simulink model "gm_uz_mlp_three_layer"  (R2021a)
settings: Solver=FixedStepDiscrete  StartTime=0.0  StopTime=5000  RelTol=1e-3
undefined symbols (not defined in the file or in its folder): nn, nn_data_type_max, numInput, numOut
libraries: hdlsllib x94, simulink x85
(part 3 of 4)

== system gm_uz_mlp_three_layer/uz_mlp_three_layer/reluLayer_8Parallel/MAC7 ==
  rd_addr : Inport  OutDataTypeStr=fixdt(0, 10, 0)  PortDimensions=1  SampleTime=1
  b : Inport  Port=2  OutDataTypeStr=fixdt(1, 32, 14)  PortDimensions=1  SampleTime=1
  axi_signals : Inport  Port=3  SampleTime=1
  fromStateMachine : Inport  Port=4  SampleTime=1
  AND : Logic  IconShape=distinctive  AllPortsSameDT=off  OutDataTypeStr=boolean
  AND1 : Logic  IconShape=distinctive  AllPortsSameDT=off  OutDataTypeStr=boolean
  Bus Selector : BusSelector  OutputSignals=axi_weightData,axi_weightAddr,axi_weightsWriteEnable,axi_biasData,axi_biasAddr,axi_biasWriteEnable,axi_layerNr
  Bus Selector1 : BusSelector  OutputSignals=endin,validIn,startin,mac_counter,write_enable,n_perceptron
  Compare To Constant : simulink/Logic and Bit Operations/Compare To Constant  relop===  const=ParallelNr  OutDataTypeStr=boolean
  Compare To Constant1 : simulink/Logic and Bit Operations/Compare To Constant  relop===  const=ParallelNr  OutDataTypeStr=boolean
  Compare To Constant2 : simulink/Logic and Bit Operations/Compare To Constant  relop===  const=LayerNr  OutDataTypeStr=boolean
  Constant : Constant  Value=nStart  OutDataTypeStr=Inherit: Inherit via back propagation  SampleTime=-1
  Dual Port RAM System1 : hdlsllib/HDL RAMs/Dual Port RAM System  RAMType=Simple dual port  WriteOutputValue=New data  RAMInitialValue=[layer.bias(nStart:nEnd);zeros(1024-length(layer.bias(nStart:nEnd)),1)]  SimulateUsing=Code generation
      settings: SourceProductBaseCode=SL
  Dual Port RAM System2 : hdlsllib/HDL RAMs/Dual Port RAM System  RAMType=Simple dual port  WriteOutputValue=New data  RAMInitialValue=[0]  SimulateUsing=Code generation
      settings: SourceProductBaseCode=SL
  Dual Port RAM System3 : hdlsllib/HDL RAMs/Dual Port RAM System  RAMType=Simple dual port  WriteOutputValue=New data  RAMInitialValue=[0;reshape(layer.weights(:,nStart:nEnd),[],1);zeros(1023-length(reshape(layer.weights(:,nStart:nEnd),[],1)),1)]  SimulateUsing=Code generation
      settings: SourceProductBaseCode=SL
  Gain : Gain  Gain=size(layer.weights(:,nStart:nEnd),1)  OutDataTypeStr=Inherit: Same as input
  Multiply-Accumulate1 : hdlsllib/HDL Operations/Multiply-Accumulate  opMode=Streaming - using Start and End ports  initValueSetting=Dialog  initValue=0  initValueSetting2=Input port  initValue2=0  initValueSetting3=Dialog  initValue3=0  num_samples=2  RndMeth2=Floor  RndMeth3=Floor  datatype2=fixdt(1,32,14)  datatype3=Inherit: Inherit via back propagation  validOut=on  endInandOut=on  startOut=on  countOut=on  dim=-1  DoSatur=off  parallel=off
      settings: SourceProductBaseCode=SL
  Saturation1 : Saturate  UpperLimit=nn_data_type_max  LowerLimit=0
  Sum : Sum  Inputs=|++  OutDataTypeStr=Inherit: Same as first input
  Sum1 : Sum  Inputs=|++  OutDataTypeStr=Inherit: Same as first input
  Terminator : Terminator
  rd_dout : Outport  SampleTime=1
  startOut : Outport  Port=2  SampleTime=1
  endOut : Outport  Port=3  SampleTime=1
  wires:
  rd_addr/1 -> Dual Port RAM System2/4
  b/1 -> Multiply-Accumulate1/2
  axi_signals/1 -> Bus Selector/1
  fromStateMachine/1 -> Bus Selector1/1
  AND/1 -> Dual Port RAM System3/3
  AND1/1 -> Dual Port RAM System1/3
  Bus Selector/1 -> Dual Port RAM System3/1
  Bus Selector/2 -> Dual Port RAM System3/2
  Bus Selector/3 -> Compare To Constant/1
  Bus Selector/4 -> Dual Port RAM System1/1
  Bus Selector/5 -> Dual Port RAM System1/2
  Bus Selector/6 -> Compare To Constant1/1
  Bus Selector/7 -> Compare To Constant2/1
  Bus Selector1/1 -> Multiply-Accumulate1/4
  Bus Selector1/2 -> Multiply-Accumulate1/5
  Bus Selector1/3 -> Multiply-Accumulate1/3
  Bus Selector1/4 -> Sum1/2
  Bus Selector1/5 -> Dual Port RAM System2/3
  Bus Selector1/6 -> Sum/1, Gain/1, Dual Port RAM System1/4
  Compare To Constant/1 -> AND/1
  Compare To Constant1/1 -> AND1/1
  Compare To Constant2/1 -> AND1/2, AND/2
  Constant/1 -> Sum/2
  Dual Port RAM System1/1 -> Multiply-Accumulate1/6
  Dual Port RAM System2/1 -> rd_dout/1
  Dual Port RAM System3/1 -> Multiply-Accumulate1/1
  Gain/1 -> Sum1/1
  Multiply-Accumulate1/1 -> Saturation1/1
  Multiply-Accumulate1/2 -> startOut/1
  Multiply-Accumulate1/3 -> endOut/1
  Multiply-Accumulate1/4 -> Terminator/1
  Saturation1/1 -> Dual Port RAM System2/1
  Sum/1 -> Dual Port RAM System2/2
  Sum1/1 -> Dual Port RAM System3/4

== system gm_uz_mlp_three_layer/uz_mlp_three_layer/reluLayer_8Parallel/MATLAB Function1 ==
  readAddr : Inport  OutDataTypeStr=fixdt(0, 10, 0)  PortDimensions=1  SampleTime=1
  MATLAB Function1 : MATLAB Function  TreatAsAtomicUnit=on
  y : Outport  SampleTime=1
  wires:
  readAddr/1 -> MATLAB Function1/1(readAddr)
  MATLAB Function1/1(y) -> y/1

== system gm_uz_mlp_three_layer/uz_mlp_three_layer/reluLayer_8Parallel/StateMachines1 ==
  triggerCalc : Inport  OutDataTypeStr=boolean  SampleTime=1
  mac_startOut : Inport  Port=2  OutDataTypeStr=boolean  SampleTime=1
  end_out : Inport  Port=3  OutDataTypeStr=boolean  SampleTime=1
  Bus Creator : BusCreator  Inputs=6
  Compare To Constant : simulink/Logic and Bit Operations/Compare To Constant  relop===  const=layer.weight_dimension(1)  OutDataTypeStr=boolean
  Compare To Constant1 : simulink/Logic and Bit Operations/Compare To Constant  relop===  const=layer.weight_dimension(2)/ParallelDSP-1  OutDataTypeStr=boolean
  Delay2 : Delay  DelayLength=1
  Delay3 : Delay  DelayLength=1
  Delay4 : Delay  DelayLength=1
  Detect Rise Positive : simulink/Logic and Bit Operations/Detect Rise Positive  vinit=0  OutDataTypeStr=boolean
  index_counter : hdlsllib/Sources/HDL Counter  CountType=Count limited  CountInit=1  CountStep=1  CountMax=layer.weight_dimension(1)  CountFromType=Initial value  CountFrom=1  CountResetPort=on  CountLoadPort=off  CountEnbPort=on  CountDirPort=off  CountHitOutputPort=off  CountDataType=Unsigned  CountWordLen=10  CountFracLen=0  CountSampTime=1
  layer_control : Subsystem
  mac_control : Subsystem
  perceptron_counter1 : hdlsllib/Sources/HDL Counter  CountType=Count limited  CountInit=0  CountStep=1  CountMax=layer.weight_dimension(2)/ParallelDSP-1  CountFromType=Initial value  CountFrom=0  CountResetPort=on  CountLoadPort=off  CountEnbPort=on  CountDirPort=off  CountHitOutputPort=off  CountDataType=Unsigned  CountWordLen=10  CountFracLen=0  CountSampTime=1
  mac_counter : Outport  SampleTime=1
  layer_rdy : Outport  Port=2  SampleTime=1
  layer_finished : Outport  Port=3  SampleTime=1
  toMac : Outport  Port=4  SampleTime=1
  wires:
  triggerCalc/1 -> Detect Rise Positive/1
  mac_startOut/1 -> mac_control/5(mac_startOut)
  end_out/1 -> Delay3/1, mac_control/3(end_out)
  Bus Creator/1 -> toMac/1
  Compare To Constant/1 -> mac_control/2(counter_finished)
  Compare To Constant1/1 -> layer_control/3(cnt_finished)
  Delay2/1 -> Compare To Constant/1
  Delay3/1 -> mac_control/4(end_out_delay)
  Delay4/1 -> layer_control/2(mac_ready)
  Detect Rise Positive/1 -> layer_control/1(ext_enable)
  index_counter/1 -> Bus Creator/4, Delay2/1, mac_counter/1  "mac_counter"
  layer_control/1(enable_mac) -> mac_control/1(external_enable)
  layer_control/2(layer_rdy) -> layer_rdy/1
  layer_control/3(cnt_enable) -> perceptron_counter1/2
  layer_control/4(counter_rest) -> perceptron_counter1/1
  layer_control/5(layer_finished) -> layer_finished/1
  mac_control/1(index_counter_enb) -> index_counter/2
  mac_control/2(mac_startIn) -> Bus Creator/3  "startin"
  mac_control/3(mac_endIn) -> Bus Creator/1  "endin"
  mac_control/4(mac_validIn) -> Bus Creator/2  "validIn"
  mac_control/5(index_counter_rst) -> index_counter/1
  mac_control/6(write_ram) -> Bus Creator/5  "write_enable"
  mac_control/7(mac_ready) -> Delay4/1
  perceptron_counter1/1 -> Compare To Constant1/1, Bus Creator/6  "n_perceptron"

== system gm_uz_mlp_three_layer/uz_mlp_three_layer/reluLayer_8Parallel1/MAC ==
  rd_addr : Inport  OutDataTypeStr=fixdt(0, 10, 0)  PortDimensions=1  SampleTime=1
  b : Inport  Port=2  OutDataTypeStr=fixdt(1, 32, 14)  PortDimensions=1  SampleTime=1
  axi_signals : Inport  Port=3  SampleTime=1
  fromStateMachine : Inport  Port=4  SampleTime=1
  AND : Logic  IconShape=distinctive  AllPortsSameDT=off  OutDataTypeStr=boolean
  AND1 : Logic  IconShape=distinctive  AllPortsSameDT=off  OutDataTypeStr=boolean
  Bus Selector : BusSelector  OutputSignals=axi_weightData,axi_weightAddr,axi_weightsWriteEnable,axi_biasData,axi_biasAddr,axi_biasWriteEnable,axi_layerNr
  Bus Selector1 : BusSelector  OutputSignals=endin,validIn,startin,mac_counter,write_enable,n_perceptron
  Compare To Constant : simulink/Logic and Bit Operations/Compare To Constant  relop===  const=ParallelNr  OutDataTypeStr=boolean
  Compare To Constant1 : simulink/Logic and Bit Operations/Compare To Constant  relop===  const=ParallelNr  OutDataTypeStr=boolean
  Compare To Constant2 : simulink/Logic and Bit Operations/Compare To Constant  relop===  const=LayerNr  OutDataTypeStr=boolean
  Constant : Constant  Value=nStart  OutDataTypeStr=Inherit: Inherit via back propagation  SampleTime=-1
  Dual Port RAM System1 : hdlsllib/HDL RAMs/Dual Port RAM System  RAMType=Simple dual port  WriteOutputValue=New data  RAMInitialValue=[layer.bias(nStart:nEnd);zeros(1024-length(layer.bias(nStart:nEnd)),1)]  SimulateUsing=Code generation
      settings: SourceProductBaseCode=SL
  Dual Port RAM System2 : hdlsllib/HDL RAMs/Dual Port RAM System  RAMType=Simple dual port  WriteOutputValue=New data  RAMInitialValue=[0]  SimulateUsing=Code generation
      settings: SourceProductBaseCode=SL
  Dual Port RAM System3 : hdlsllib/HDL RAMs/Dual Port RAM System  RAMType=Simple dual port  WriteOutputValue=New data  RAMInitialValue=[0;reshape(layer.weights(:,nStart:nEnd),[],1);zeros(1023-length(reshape(layer.weights(:,nStart:nEnd),[],1)),1)]  SimulateUsing=Code generation
      settings: SourceProductBaseCode=SL
  Gain : Gain  Gain=size(layer.weights(:,nStart:nEnd),1)  OutDataTypeStr=Inherit: Same as input
  Multiply-Accumulate1 : hdlsllib/HDL Operations/Multiply-Accumulate  opMode=Streaming - using Start and End ports  initValueSetting=Dialog  initValue=0  initValueSetting2=Input port  initValue2=0  initValueSetting3=Dialog  initValue3=0  num_samples=2  RndMeth2=Floor  RndMeth3=Floor  datatype2=fixdt(1,32,14)  datatype3=Inherit: Inherit via back propagation  validOut=on  endInandOut=on  startOut=on  countOut=on  dim=-1  DoSatur=off  parallel=off
      settings: SourceProductBaseCode=SL
  Saturation1 : Saturate  UpperLimit=nn_data_type_max  LowerLimit=0
  Sum : Sum  Inputs=|++  OutDataTypeStr=Inherit: Same as first input
  Sum1 : Sum  Inputs=|++  OutDataTypeStr=Inherit: Same as first input
  Terminator : Terminator
  rd_dout : Outport  SampleTime=1
  startOut : Outport  Port=2  SampleTime=1
  endOut : Outport  Port=3  SampleTime=1
  wires:
  rd_addr/1 -> Dual Port RAM System2/4
  b/1 -> Multiply-Accumulate1/2
  axi_signals/1 -> Bus Selector/1
  fromStateMachine/1 -> Bus Selector1/1
  AND/1 -> Dual Port RAM System3/3
  AND1/1 -> Dual Port RAM System1/3
  Bus Selector/1 -> Dual Port RAM System3/1
  Bus Selector/2 -> Dual Port RAM System3/2
  Bus Selector/3 -> Compare To Constant/1
  Bus Selector/4 -> Dual Port RAM System1/1
  Bus Selector/5 -> Dual Port RAM System1/2
  Bus Selector/6 -> Compare To Constant1/1
  Bus Selector/7 -> Compare To Constant2/1
  Bus Selector1/1 -> Multiply-Accumulate1/4
  Bus Selector1/2 -> Multiply-Accumulate1/5
  Bus Selector1/3 -> Multiply-Accumulate1/3
  Bus Selector1/4 -> Sum1/2
  Bus Selector1/5 -> Dual Port RAM System2/3
  Bus Selector1/6 -> Sum/1, Gain/1, Dual Port RAM System1/4
  Compare To Constant/1 -> AND/1
  Compare To Constant1/1 -> AND1/1
  Compare To Constant2/1 -> AND1/2, AND/2
  Constant/1 -> Sum/2
  Dual Port RAM System1/1 -> Multiply-Accumulate1/6
  Dual Port RAM System2/1 -> rd_dout/1
  Dual Port RAM System3/1 -> Multiply-Accumulate1/1
  Gain/1 -> Sum1/1
  Multiply-Accumulate1/1 -> Saturation1/1
  Multiply-Accumulate1/2 -> startOut/1
  Multiply-Accumulate1/3 -> endOut/1
  Multiply-Accumulate1/4 -> Terminator/1
  Saturation1/1 -> Dual Port RAM System2/1
  Sum/1 -> Dual Port RAM System2/2
  Sum1/1 -> Dual Port RAM System3/4

== system gm_uz_mlp_three_layer/uz_mlp_three_layer/reluLayer_8Parallel1/MAC1 ==
  rd_addr : Inport  OutDataTypeStr=fixdt(0, 10, 0)  PortDimensions=1  SampleTime=1
  b : Inport  Port=2  OutDataTypeStr=fixdt(1, 32, 14)  PortDimensions=1  SampleTime=1
  axi_signals : Inport  Port=3  SampleTime=1
  fromStateMachine : Inport  Port=4  SampleTime=1
  AND : Logic  IconShape=distinctive  AllPortsSameDT=off  OutDataTypeStr=boolean
  AND1 : Logic  IconShape=distinctive  AllPortsSameDT=off  OutDataTypeStr=boolean
  Bus Selector : BusSelector  OutputSignals=axi_weightData,axi_weightAddr,axi_weightsWriteEnable,axi_biasData,axi_biasAddr,axi_biasWriteEnable,axi_layerNr
  Bus Selector1 : BusSelector  OutputSignals=endin,validIn,startin,mac_counter,write_enable,n_perceptron
  Compare To Constant : simulink/Logic and Bit Operations/Compare To Constant  relop===  const=ParallelNr  OutDataTypeStr=boolean
  Compare To Constant1 : simulink/Logic and Bit Operations/Compare To Constant  relop===  const=ParallelNr  OutDataTypeStr=boolean
  Compare To Constant2 : simulink/Logic and Bit Operations/Compare To Constant  relop===  const=LayerNr  OutDataTypeStr=boolean
  Constant : Constant  Value=nStart  OutDataTypeStr=Inherit: Inherit via back propagation  SampleTime=-1
  Dual Port RAM System1 : hdlsllib/HDL RAMs/Dual Port RAM System  RAMType=Simple dual port  WriteOutputValue=New data  RAMInitialValue=[layer.bias(nStart:nEnd);zeros(1024-length(layer.bias(nStart:nEnd)),1)]  SimulateUsing=Code generation
      settings: SourceProductBaseCode=SL
  Dual Port RAM System2 : hdlsllib/HDL RAMs/Dual Port RAM System  RAMType=Simple dual port  WriteOutputValue=New data  RAMInitialValue=[0]  SimulateUsing=Code generation
      settings: SourceProductBaseCode=SL
  Dual Port RAM System3 : hdlsllib/HDL RAMs/Dual Port RAM System  RAMType=Simple dual port  WriteOutputValue=New data  RAMInitialValue=[0;reshape(layer.weights(:,nStart:nEnd),[],1);zeros(1023-length(reshape(layer.weights(:,nStart:nEnd),[],1)),1)]  SimulateUsing=Code generation
      settings: SourceProductBaseCode=SL
  Gain : Gain  Gain=size(layer.weights(:,nStart:nEnd),1)  OutDataTypeStr=Inherit: Same as input
  Multiply-Accumulate1 : hdlsllib/HDL Operations/Multiply-Accumulate  opMode=Streaming - using Start and End ports  initValueSetting=Dialog  initValue=0  initValueSetting2=Input port  initValue2=0  initValueSetting3=Dialog  initValue3=0  num_samples=2  RndMeth2=Floor  RndMeth3=Floor  datatype2=fixdt(1,32,14)  datatype3=Inherit: Inherit via back propagation  validOut=on  endInandOut=on  startOut=on  countOut=on  dim=-1  DoSatur=off  parallel=off
      settings: SourceProductBaseCode=SL
  Saturation1 : Saturate  UpperLimit=nn_data_type_max  LowerLimit=0
  Sum : Sum  Inputs=|++  OutDataTypeStr=Inherit: Same as first input
  Sum1 : Sum  Inputs=|++  OutDataTypeStr=Inherit: Same as first input
  Terminator : Terminator
  rd_dout : Outport  SampleTime=1
  startOut : Outport  Port=2  SampleTime=1
  endOut : Outport  Port=3  SampleTime=1
  wires:
  rd_addr/1 -> Dual Port RAM System2/4
  b/1 -> Multiply-Accumulate1/2
  axi_signals/1 -> Bus Selector/1
  fromStateMachine/1 -> Bus Selector1/1
  AND/1 -> Dual Port RAM System3/3
  AND1/1 -> Dual Port RAM System1/3
  Bus Selector/1 -> Dual Port RAM System3/1
  Bus Selector/2 -> Dual Port RAM System3/2
  Bus Selector/3 -> Compare To Constant/1
  Bus Selector/4 -> Dual Port RAM System1/1
  Bus Selector/5 -> Dual Port RAM System1/2
  Bus Selector/6 -> Compare To Constant1/1
  Bus Selector/7 -> Compare To Constant2/1
  Bus Selector1/1 -> Multiply-Accumulate1/4
  Bus Selector1/2 -> Multiply-Accumulate1/5
  Bus Selector1/3 -> Multiply-Accumulate1/3
  Bus Selector1/4 -> Sum1/2
  Bus Selector1/5 -> Dual Port RAM System2/3
  Bus Selector1/6 -> Sum/1, Gain/1, Dual Port RAM System1/4
  Compare To Constant/1 -> AND/1
  Compare To Constant1/1 -> AND1/1
  Compare To Constant2/1 -> AND1/2, AND/2
  Constant/1 -> Sum/2
  Dual Port RAM System1/1 -> Multiply-Accumulate1/6
  Dual Port RAM System2/1 -> rd_dout/1
  Dual Port RAM System3/1 -> Multiply-Accumulate1/1
  Gain/1 -> Sum1/1
  Multiply-Accumulate1/1 -> Saturation1/1
  Multiply-Accumulate1/2 -> startOut/1
  Multiply-Accumulate1/3 -> endOut/1
  Multiply-Accumulate1/4 -> Terminator/1
  Saturation1/1 -> Dual Port RAM System2/1
  Sum/1 -> Dual Port RAM System2/2
  Sum1/1 -> Dual Port RAM System3/4

== system gm_uz_mlp_three_layer/uz_mlp_three_layer/reluLayer_8Parallel1/MAC2 ==
  rd_addr : Inport  OutDataTypeStr=fixdt(0, 10, 0)  PortDimensions=1  SampleTime=1
  b : Inport  Port=2  OutDataTypeStr=fixdt(1, 32, 14)  PortDimensions=1  SampleTime=1
  axi_signals : Inport  Port=3  SampleTime=1
  fromStateMachine : Inport  Port=4  SampleTime=1
  AND : Logic  IconShape=distinctive  AllPortsSameDT=off  OutDataTypeStr=boolean
  AND1 : Logic  IconShape=distinctive  AllPortsSameDT=off  OutDataTypeStr=boolean
  Bus Selector : BusSelector  OutputSignals=axi_weightData,axi_weightAddr,axi_weightsWriteEnable,axi_biasData,axi_biasAddr,axi_biasWriteEnable,axi_layerNr
  Bus Selector1 : BusSelector  OutputSignals=endin,validIn,startin,mac_counter,write_enable,n_perceptron
  Compare To Constant : simulink/Logic and Bit Operations/Compare To Constant  relop===  const=ParallelNr  OutDataTypeStr=boolean
  Compare To Constant1 : simulink/Logic and Bit Operations/Compare To Constant  relop===  const=ParallelNr  OutDataTypeStr=boolean
  Compare To Constant2 : simulink/Logic and Bit Operations/Compare To Constant  relop===  const=LayerNr  OutDataTypeStr=boolean
  Constant : Constant  Value=nStart  OutDataTypeStr=Inherit: Inherit via back propagation  SampleTime=-1
  Dual Port RAM System1 : hdlsllib/HDL RAMs/Dual Port RAM System  RAMType=Simple dual port  WriteOutputValue=New data  RAMInitialValue=[layer.bias(nStart:nEnd);zeros(1024-length(layer.bias(nStart:nEnd)),1)]  SimulateUsing=Code generation
      settings: SourceProductBaseCode=SL
  Dual Port RAM System2 : hdlsllib/HDL RAMs/Dual Port RAM System  RAMType=Simple dual port  WriteOutputValue=New data  RAMInitialValue=[0]  SimulateUsing=Code generation
      settings: SourceProductBaseCode=SL
  Dual Port RAM System3 : hdlsllib/HDL RAMs/Dual Port RAM System  RAMType=Simple dual port  WriteOutputValue=New data  RAMInitialValue=[0;reshape(layer.weights(:,nStart:nEnd),[],1);zeros(1023-length(reshape(layer.weights(:,nStart:nEnd),[],1)),1)]  SimulateUsing=Code generation
      settings: SourceProductBaseCode=SL
  Gain : Gain  Gain=size(layer.weights(:,nStart:nEnd),1)  OutDataTypeStr=Inherit: Same as input
  Multiply-Accumulate1 : hdlsllib/HDL Operations/Multiply-Accumulate  opMode=Streaming - using Start and End ports  initValueSetting=Dialog  initValue=0  initValueSetting2=Input port  initValue2=0  initValueSetting3=Dialog  initValue3=0  num_samples=2  RndMeth2=Floor  RndMeth3=Floor  datatype2=fixdt(1,32,14)  datatype3=Inherit: Inherit via back propagation  validOut=on  endInandOut=on  startOut=on  countOut=on  dim=-1  DoSatur=off  parallel=off
      settings: SourceProductBaseCode=SL
  Saturation1 : Saturate  UpperLimit=nn_data_type_max  LowerLimit=0
  Sum : Sum  Inputs=|++  OutDataTypeStr=Inherit: Same as first input
  Sum1 : Sum  Inputs=|++  OutDataTypeStr=Inherit: Same as first input
  Terminator : Terminator
  rd_dout : Outport  SampleTime=1
  startOut : Outport  Port=2  SampleTime=1
  endOut : Outport  Port=3  SampleTime=1
  wires:
  rd_addr/1 -> Dual Port RAM System2/4
  b/1 -> Multiply-Accumulate1/2
  axi_signals/1 -> Bus Selector/1
  fromStateMachine/1 -> Bus Selector1/1
  AND/1 -> Dual Port RAM System3/3
  AND1/1 -> Dual Port RAM System1/3
  Bus Selector/1 -> Dual Port RAM System3/1
  Bus Selector/2 -> Dual Port RAM System3/2
  Bus Selector/3 -> Compare To Constant/1
  Bus Selector/4 -> Dual Port RAM System1/1
  Bus Selector/5 -> Dual Port RAM System1/2
  Bus Selector/6 -> Compare To Constant1/1
  Bus Selector/7 -> Compare To Constant2/1
  Bus Selector1/1 -> Multiply-Accumulate1/4
  Bus Selector1/2 -> Multiply-Accumulate1/5
  Bus Selector1/3 -> Multiply-Accumulate1/3
  Bus Selector1/4 -> Sum1/2
  Bus Selector1/5 -> Dual Port RAM System2/3
  Bus Selector1/6 -> Sum/1, Gain/1, Dual Port RAM System1/4
  Compare To Constant/1 -> AND/1
  Compare To Constant1/1 -> AND1/1
  Compare To Constant2/1 -> AND1/2, AND/2
  Constant/1 -> Sum/2
  Dual Port RAM System1/1 -> Multiply-Accumulate1/6
  Dual Port RAM System2/1 -> rd_dout/1
  Dual Port RAM System3/1 -> Multiply-Accumulate1/1
  Gain/1 -> Sum1/1
  Multiply-Accumulate1/1 -> Saturation1/1
  Multiply-Accumulate1/2 -> startOut/1
  Multiply-Accumulate1/3 -> endOut/1
  Multiply-Accumulate1/4 -> Terminator/1
  Saturation1/1 -> Dual Port RAM System2/1
  Sum/1 -> Dual Port RAM System2/2
  Sum1/1 -> Dual Port RAM System3/4

== system gm_uz_mlp_three_layer/uz_mlp_three_layer/reluLayer_8Parallel1/MAC3 ==
  rd_addr : Inport  OutDataTypeStr=fixdt(0, 10, 0)  PortDimensions=1  SampleTime=1
  b : Inport  Port=2  OutDataTypeStr=fixdt(1, 32, 14)  PortDimensions=1  SampleTime=1
  axi_signals : Inport  Port=3  SampleTime=1
  fromStateMachine : Inport  Port=4  SampleTime=1
  AND : Logic  IconShape=distinctive  AllPortsSameDT=off  OutDataTypeStr=boolean
  AND1 : Logic  IconShape=distinctive  AllPortsSameDT=off  OutDataTypeStr=boolean
  Bus Selector : BusSelector  OutputSignals=axi_weightData,axi_weightAddr,axi_weightsWriteEnable,axi_biasData,axi_biasAddr,axi_biasWriteEnable,axi_layerNr
  Bus Selector1 : BusSelector  OutputSignals=endin,validIn,startin,mac_counter,write_enable,n_perceptron
  Compare To Constant : simulink/Logic and Bit Operations/Compare To Constant  relop===  const=ParallelNr  OutDataTypeStr=boolean
  Compare To Constant1 : simulink/Logic and Bit Operations/Compare To Constant  relop===  const=ParallelNr  OutDataTypeStr=boolean
  Compare To Constant2 : simulink/Logic and Bit Operations/Compare To Constant  relop===  const=LayerNr  OutDataTypeStr=boolean
  Constant : Constant  Value=nStart  OutDataTypeStr=Inherit: Inherit via back propagation  SampleTime=-1
  Dual Port RAM System1 : hdlsllib/HDL RAMs/Dual Port RAM System  RAMType=Simple dual port  WriteOutputValue=New data  RAMInitialValue=[layer.bias(nStart:nEnd);zeros(1024-length(layer.bias(nStart:nEnd)),1)]  SimulateUsing=Code generation
      settings: SourceProductBaseCode=SL
  Dual Port RAM System2 : hdlsllib/HDL RAMs/Dual Port RAM System  RAMType=Simple dual port  WriteOutputValue=New data  RAMInitialValue=[0]  SimulateUsing=Code generation
      settings: SourceProductBaseCode=SL
  Dual Port RAM System3 : hdlsllib/HDL RAMs/Dual Port RAM System  RAMType=Simple dual port  WriteOutputValue=New data  RAMInitialValue=[0;reshape(layer.weights(:,nStart:nEnd),[],1);zeros(1023-length(reshape(layer.weights(:,nStart:nEnd),[],1)),1)]  SimulateUsing=Code generation
      settings: SourceProductBaseCode=SL
  Gain : Gain  Gain=size(layer.weights(:,nStart:nEnd),1)  OutDataTypeStr=Inherit: Same as input
  Multiply-Accumulate1 : hdlsllib/HDL Operations/Multiply-Accumulate  opMode=Streaming - using Start and End ports  initValueSetting=Dialog  initValue=0  initValueSetting2=Input port  initValue2=0  initValueSetting3=Dialog  initValue3=0  num_samples=2  RndMeth2=Floor  RndMeth3=Floor  datatype2=fixdt(1,32,14)  datatype3=Inherit: Inherit via back propagation  validOut=on  endInandOut=on  startOut=on  countOut=on  dim=-1  DoSatur=off  parallel=off
      settings: SourceProductBaseCode=SL
  Saturation1 : Saturate  UpperLimit=nn_data_type_max  LowerLimit=0
  Sum : Sum  Inputs=|++  OutDataTypeStr=Inherit: Same as first input
  Sum1 : Sum  Inputs=|++  OutDataTypeStr=Inherit: Same as first input
  Terminator : Terminator
  rd_dout : Outport  SampleTime=1
  startOut : Outport  Port=2  SampleTime=1
  endOut : Outport  Port=3  SampleTime=1
  wires:
  rd_addr/1 -> Dual Port RAM System2/4
  b/1 -> Multiply-Accumulate1/2
  axi_signals/1 -> Bus Selector/1
  fromStateMachine/1 -> Bus Selector1/1
  AND/1 -> Dual Port RAM System3/3
  AND1/1 -> Dual Port RAM System1/3
  Bus Selector/1 -> Dual Port RAM System3/1
  Bus Selector/2 -> Dual Port RAM System3/2
  Bus Selector/3 -> Compare To Constant/1
  Bus Selector/4 -> Dual Port RAM System1/1
  Bus Selector/5 -> Dual Port RAM System1/2
  Bus Selector/6 -> Compare To Constant1/1
  Bus Selector/7 -> Compare To Constant2/1
  Bus Selector1/1 -> Multiply-Accumulate1/4
  Bus Selector1/2 -> Multiply-Accumulate1/5
  Bus Selector1/3 -> Multiply-Accumulate1/3
  Bus Selector1/4 -> Sum1/2
  Bus Selector1/5 -> Dual Port RAM System2/3
  Bus Selector1/6 -> Sum/1, Gain/1, Dual Port RAM System1/4
  Compare To Constant/1 -> AND/1
  Compare To Constant1/1 -> AND1/1
  Compare To Constant2/1 -> AND1/2, AND/2
  Constant/1 -> Sum/2
  Dual Port RAM System1/1 -> Multiply-Accumulate1/6
  Dual Port RAM System2/1 -> rd_dout/1
  Dual Port RAM System3/1 -> Multiply-Accumulate1/1
  Gain/1 -> Sum1/1
  Multiply-Accumulate1/1 -> Saturation1/1
  Multiply-Accumulate1/2 -> startOut/1
  Multiply-Accumulate1/3 -> endOut/1
  Multiply-Accumulate1/4 -> Terminator/1
  Saturation1/1 -> Dual Port RAM System2/1
  Sum/1 -> Dual Port RAM System2/2
  Sum1/1 -> Dual Port RAM System3/4

== system gm_uz_mlp_three_layer/uz_mlp_three_layer/reluLayer_8Parallel1/MAC4 ==
  rd_addr : Inport  OutDataTypeStr=fixdt(0, 10, 0)  PortDimensions=1  SampleTime=1
  b : Inport  Port=2  OutDataTypeStr=fixdt(1, 32, 14)  PortDimensions=1  SampleTime=1
  axi_signals : Inport  Port=3  SampleTime=1
  fromStateMachine : Inport  Port=4  SampleTime=1
  AND : Logic  IconShape=distinctive  AllPortsSameDT=off  OutDataTypeStr=boolean
  AND1 : Logic  IconShape=distinctive  AllPortsSameDT=off  OutDataTypeStr=boolean
  Bus Selector : BusSelector  OutputSignals=axi_weightData,axi_weightAddr,axi_weightsWriteEnable,axi_biasData,axi_biasAddr,axi_biasWriteEnable,axi_layerNr
  Bus Selector1 : BusSelector  OutputSignals=endin,validIn,startin,mac_counter,write_enable,n_perceptron
  Compare To Constant : simulink/Logic and Bit Operations/Compare To Constant  relop===  const=ParallelNr  OutDataTypeStr=boolean
  Compare To Constant1 : simulink/Logic and Bit Operations/Compare To Constant  relop===  const=ParallelNr  OutDataTypeStr=boolean
  Compare To Constant2 : simulink/Logic and Bit Operations/Compare To Constant  relop===  const=LayerNr  OutDataTypeStr=boolean
  Constant : Constant  Value=nStart  OutDataTypeStr=Inherit: Inherit via back propagation  SampleTime=-1
  Dual Port RAM System1 : hdlsllib/HDL RAMs/Dual Port RAM System  RAMType=Simple dual port  WriteOutputValue=New data  RAMInitialValue=[layer.bias(nStart:nEnd);zeros(1024-length(layer.bias(nStart:nEnd)),1)]  SimulateUsing=Code generation
      settings: SourceProductBaseCode=SL
  Dual Port RAM System2 : hdlsllib/HDL RAMs/Dual Port RAM System  RAMType=Simple dual port  WriteOutputValue=New data  RAMInitialValue=[0]  SimulateUsing=Code generation
      settings: SourceProductBaseCode=SL
  Dual Port RAM System3 : hdlsllib/HDL RAMs/Dual Port RAM System  RAMType=Simple dual port  WriteOutputValue=New data  RAMInitialValue=[0;reshape(layer.weights(:,nStart:nEnd),[],1);zeros(1023-length(reshape(layer.weights(:,nStart:nEnd),[],1)),1)]  SimulateUsing=Code generation
      settings: SourceProductBaseCode=SL
  Gain : Gain  Gain=size(layer.weights(:,nStart:nEnd),1)  OutDataTypeStr=Inherit: Same as input
  Multiply-Accumulate1 : hdlsllib/HDL Operations/Multiply-Accumulate  opMode=Streaming - using Start and End ports  initValueSetting=Dialog  initValue=0  initValueSetting2=Input port  initValue2=0  initValueSetting3=Dialog  initValue3=0  num_samples=2  RndMeth2=Floor  RndMeth3=Floor  datatype2=fixdt(1,32,14)  datatype3=Inherit: Inherit via back propagation  validOut=on  endInandOut=on  startOut=on  countOut=on  dim=-1  DoSatur=off  parallel=off
      settings: SourceProductBaseCode=SL
  Saturation1 : Saturate  UpperLimit=nn_data_type_max  LowerLimit=0
  Sum : Sum  Inputs=|++  OutDataTypeStr=Inherit: Same as first input
  Sum1 : Sum  Inputs=|++  OutDataTypeStr=Inherit: Same as first input
  Terminator : Terminator
  rd_dout : Outport  SampleTime=1
  startOut : Outport  Port=2  SampleTime=1
  endOut : Outport  Port=3  SampleTime=1
  wires:
  rd_addr/1 -> Dual Port RAM System2/4
  b/1 -> Multiply-Accumulate1/2
  axi_signals/1 -> Bus Selector/1
  fromStateMachine/1 -> Bus Selector1/1
  AND/1 -> Dual Port RAM System3/3
  AND1/1 -> Dual Port RAM System1/3
  Bus Selector/1 -> Dual Port RAM System3/1
  Bus Selector/2 -> Dual Port RAM System3/2
  Bus Selector/3 -> Compare To Constant/1
  Bus Selector/4 -> Dual Port RAM System1/1
  Bus Selector/5 -> Dual Port RAM System1/2
  Bus Selector/6 -> Compare To Constant1/1
  Bus Selector/7 -> Compare To Constant2/1
  Bus Selector1/1 -> Multiply-Accumulate1/4
  Bus Selector1/2 -> Multiply-Accumulate1/5
  Bus Selector1/3 -> Multiply-Accumulate1/3
  Bus Selector1/4 -> Sum1/2
  Bus Selector1/5 -> Dual Port RAM System2/3
  Bus Selector1/6 -> Sum/1, Gain/1, Dual Port RAM System1/4
  Compare To Constant/1 -> AND/1
  Compare To Constant1/1 -> AND1/1
  Compare To Constant2/1 -> AND1/2, AND/2
  Constant/1 -> Sum/2
  Dual Port RAM System1/1 -> Multiply-Accumulate1/6
  Dual Port RAM System2/1 -> rd_dout/1
  Dual Port RAM System3/1 -> Multiply-Accumulate1/1
  Gain/1 -> Sum1/1
  Multiply-Accumulate1/1 -> Saturation1/1
  Multiply-Accumulate1/2 -> startOut/1
  Multiply-Accumulate1/3 -> endOut/1
  Multiply-Accumulate1/4 -> Terminator/1
  Saturation1/1 -> Dual Port RAM System2/1
  Sum/1 -> Dual Port RAM System2/2
  Sum1/1 -> Dual Port RAM System3/4

== system gm_uz_mlp_three_layer/uz_mlp_three_layer/reluLayer_8Parallel1/MAC5 ==
  rd_addr : Inport  OutDataTypeStr=fixdt(0, 10, 0)  PortDimensions=1  SampleTime=1
  b : Inport  Port=2  OutDataTypeStr=fixdt(1, 32, 14)  PortDimensions=1  SampleTime=1
  axi_signals : Inport  Port=3  SampleTime=1
  fromStateMachine : Inport  Port=4  SampleTime=1
  AND : Logic  IconShape=distinctive  AllPortsSameDT=off  OutDataTypeStr=boolean
  AND1 : Logic  IconShape=distinctive  AllPortsSameDT=off  OutDataTypeStr=boolean
  Bus Selector : BusSelector  OutputSignals=axi_weightData,axi_weightAddr,axi_weightsWriteEnable,axi_biasData,axi_biasAddr,axi_biasWriteEnable,axi_layerNr
  Bus Selector1 : BusSelector  OutputSignals=endin,validIn,startin,mac_counter,write_enable,n_perceptron
  Compare To Constant : simulink/Logic and Bit Operations/Compare To Constant  relop===  const=ParallelNr  OutDataTypeStr=boolean
  Compare To Constant1 : simulink/Logic and Bit Operations/Compare To Constant  relop===  const=ParallelNr  OutDataTypeStr=boolean
  Compare To Constant2 : simulink/Logic and Bit Operations/Compare To Constant  relop===  const=LayerNr  OutDataTypeStr=boolean
  Constant : Constant  Value=nStart  OutDataTypeStr=Inherit: Inherit via back propagation  SampleTime=-1
  Dual Port RAM System1 : hdlsllib/HDL RAMs/Dual Port RAM System  RAMType=Simple dual port  WriteOutputValue=New data  RAMInitialValue=[layer.bias(nStart:nEnd);zeros(1024-length(layer.bias(nStart:nEnd)),1)]  SimulateUsing=Code generation
      settings: SourceProductBaseCode=SL
  Dual Port RAM System2 : hdlsllib/HDL RAMs/Dual Port RAM System  RAMType=Simple dual port  WriteOutputValue=New data  RAMInitialValue=[0]  SimulateUsing=Code generation
      settings: SourceProductBaseCode=SL
  Dual Port RAM System3 : hdlsllib/HDL RAMs/Dual Port RAM System  RAMType=Simple dual port  WriteOutputValue=New data  RAMInitialValue=[0;reshape(layer.weights(:,nStart:nEnd),[],1);zeros(1023-length(reshape(layer.weights(:,nStart:nEnd),[],1)),1)]  SimulateUsing=Code generation
      settings: SourceProductBaseCode=SL
  Gain : Gain  Gain=size(layer.weights(:,nStart:nEnd),1)  OutDataTypeStr=Inherit: Same as input
  Multiply-Accumulate1 : hdlsllib/HDL Operations/Multiply-Accumulate  opMode=Streaming - using Start and End ports  initValueSetting=Dialog  initValue=0  initValueSetting2=Input port  initValue2=0  initValueSetting3=Dialog  initValue3=0  num_samples=2  RndMeth2=Floor  RndMeth3=Floor  datatype2=fixdt(1,32,14)  datatype3=Inherit: Inherit via back propagation  validOut=on  endInandOut=on  startOut=on  countOut=on  dim=-1  DoSatur=off  parallel=off
      settings: SourceProductBaseCode=SL
  Saturation1 : Saturate  UpperLimit=nn_data_type_max  LowerLimit=0
  Sum : Sum  Inputs=|++  OutDataTypeStr=Inherit: Same as first input
  Sum1 : Sum  Inputs=|++  OutDataTypeStr=Inherit: Same as first input
  Terminator : Terminator
  rd_dout : Outport  SampleTime=1
  startOut : Outport  Port=2  SampleTime=1
  endOut : Outport  Port=3  SampleTime=1
  wires:
  rd_addr/1 -> Dual Port RAM System2/4
  b/1 -> Multiply-Accumulate1/2
  axi_signals/1 -> Bus Selector/1
  fromStateMachine/1 -> Bus Selector1/1
  AND/1 -> Dual Port RAM System3/3
  AND1/1 -> Dual Port RAM System1/3
  Bus Selector/1 -> Dual Port RAM System3/1
  Bus Selector/2 -> Dual Port RAM System3/2
  Bus Selector/3 -> Compare To Constant/1
  Bus Selector/4 -> Dual Port RAM System1/1
  Bus Selector/5 -> Dual Port RAM System1/2
  Bus Selector/6 -> Compare To Constant1/1
  Bus Selector/7 -> Compare To Constant2/1
  Bus Selector1/1 -> Multiply-Accumulate1/4
  Bus Selector1/2 -> Multiply-Accumulate1/5
  Bus Selector1/3 -> Multiply-Accumulate1/3
  Bus Selector1/4 -> Sum1/2
  Bus Selector1/5 -> Dual Port RAM System2/3
  Bus Selector1/6 -> Sum/1, Gain/1, Dual Port RAM System1/4
  Compare To Constant/1 -> AND/1
  Compare To Constant1/1 -> AND1/1
  Compare To Constant2/1 -> AND1/2, AND/2
  Constant/1 -> Sum/2
  Dual Port RAM System1/1 -> Multiply-Accumulate1/6
  Dual Port RAM System2/1 -> rd_dout/1
  Dual Port RAM System3/1 -> Multiply-Accumulate1/1
  Gain/1 -> Sum1/1
  Multiply-Accumulate1/1 -> Saturation1/1
  Multiply-Accumulate1/2 -> startOut/1
  Multiply-Accumulate1/3 -> endOut/1
  Multiply-Accumulate1/4 -> Terminator/1
  Saturation1/1 -> Dual Port RAM System2/1
  Sum/1 -> Dual Port RAM System2/2
  Sum1/1 -> Dual Port RAM System3/4

== system gm_uz_mlp_three_layer/uz_mlp_three_layer/reluLayer_8Parallel1/MAC6 ==
  rd_addr : Inport  OutDataTypeStr=fixdt(0, 10, 0)  PortDimensions=1  SampleTime=1
  b : Inport  Port=2  OutDataTypeStr=fixdt(1, 32, 14)  PortDimensions=1  SampleTime=1
  axi_signals : Inport  Port=3  SampleTime=1
  fromStateMachine : Inport  Port=4  SampleTime=1
  AND : Logic  IconShape=distinctive  AllPortsSameDT=off  OutDataTypeStr=boolean
  AND1 : Logic  IconShape=distinctive  AllPortsSameDT=off  OutDataTypeStr=boolean
  Bus Selector : BusSelector  OutputSignals=axi_weightData,axi_weightAddr,axi_weightsWriteEnable,axi_biasData,axi_biasAddr,axi_biasWriteEnable,axi_layerNr
  Bus Selector1 : BusSelector  OutputSignals=endin,validIn,startin,mac_counter,write_enable,n_perceptron
  Compare To Constant : simulink/Logic and Bit Operations/Compare To Constant  relop===  const=ParallelNr  OutDataTypeStr=boolean
  Compare To Constant1 : simulink/Logic and Bit Operations/Compare To Constant  relop===  const=ParallelNr  OutDataTypeStr=boolean
  Compare To Constant2 : simulink/Logic and Bit Operations/Compare To Constant  relop===  const=LayerNr  OutDataTypeStr=boolean
  Constant : Constant  Value=nStart  OutDataTypeStr=Inherit: Inherit via back propagation  SampleTime=-1
  Dual Port RAM System1 : hdlsllib/HDL RAMs/Dual Port RAM System  RAMType=Simple dual port  WriteOutputValue=New data  RAMInitialValue=[layer.bias(nStart:nEnd);zeros(1024-length(layer.bias(nStart:nEnd)),1)]  SimulateUsing=Code generation
      settings: SourceProductBaseCode=SL
  Dual Port RAM System2 : hdlsllib/HDL RAMs/Dual Port RAM System  RAMType=Simple dual port  WriteOutputValue=New data  RAMInitialValue=[0]  SimulateUsing=Code generation
      settings: SourceProductBaseCode=SL
  Dual Port RAM System3 : hdlsllib/HDL RAMs/Dual Port RAM System  RAMType=Simple dual port  WriteOutputValue=New data  RAMInitialValue=[0;reshape(layer.weights(:,nStart:nEnd),[],1);zeros(1023-length(reshape(layer.weights(:,nStart:nEnd),[],1)),1)]  SimulateUsing=Code generation
      settings: SourceProductBaseCode=SL
  Gain : Gain  Gain=size(layer.weights(:,nStart:nEnd),1)  OutDataTypeStr=Inherit: Same as input
  Multiply-Accumulate1 : hdlsllib/HDL Operations/Multiply-Accumulate  opMode=Streaming - using Start and End ports  initValueSetting=Dialog  initValue=0  initValueSetting2=Input port  initValue2=0  initValueSetting3=Dialog  initValue3=0  num_samples=2  RndMeth2=Floor  RndMeth3=Floor  datatype2=fixdt(1,32,14)  datatype3=Inherit: Inherit via back propagation  validOut=on  endInandOut=on  startOut=on  countOut=on  dim=-1  DoSatur=off  parallel=off
      settings: SourceProductBaseCode=SL
  Saturation1 : Saturate  UpperLimit=nn_data_type_max  LowerLimit=0
  Sum : Sum  Inputs=|++  OutDataTypeStr=Inherit: Same as first input
  Sum1 : Sum  Inputs=|++  OutDataTypeStr=Inherit: Same as first input
  Terminator : Terminator
  rd_dout : Outport  SampleTime=1
  startOut : Outport  Port=2  SampleTime=1
  endOut : Outport  Port=3  SampleTime=1
  wires:
  rd_addr/1 -> Dual Port RAM System2/4
  b/1 -> Multiply-Accumulate1/2
  axi_signals/1 -> Bus Selector/1
  fromStateMachine/1 -> Bus Selector1/1
  AND/1 -> Dual Port RAM System3/3
  AND1/1 -> Dual Port RAM System1/3
  Bus Selector/1 -> Dual Port RAM System3/1
  Bus Selector/2 -> Dual Port RAM System3/2
  Bus Selector/3 -> Compare To Constant/1
  Bus Selector/4 -> Dual Port RAM System1/1
  Bus Selector/5 -> Dual Port RAM System1/2
  Bus Selector/6 -> Compare To Constant1/1
  Bus Selector/7 -> Compare To Constant2/1
  Bus Selector1/1 -> Multiply-Accumulate1/4
  Bus Selector1/2 -> Multiply-Accumulate1/5
  Bus Selector1/3 -> Multiply-Accumulate1/3
  Bus Selector1/4 -> Sum1/2
  Bus Selector1/5 -> Dual Port RAM System2/3
  Bus Selector1/6 -> Sum/1, Gain/1, Dual Port RAM System1/4
  Compare To Constant/1 -> AND/1
  Compare To Constant1/1 -> AND1/1
  Compare To Constant2/1 -> AND1/2, AND/2
  Constant/1 -> Sum/2
  Dual Port RAM System1/1 -> Multiply-Accumulate1/6
  Dual Port RAM System2/1 -> rd_dout/1
  Dual Port RAM System3/1 -> Multiply-Accumulate1/1
  Gain/1 -> Sum1/1
  Multiply-Accumulate1/1 -> Saturation1/1
  Multiply-Accumulate1/2 -> startOut/1
  Multiply-Accumulate1/3 -> endOut/1
  Multiply-Accumulate1/4 -> Terminator/1
  Saturation1/1 -> Dual Port RAM System2/1
  Sum/1 -> Dual Port RAM System2/2
  Sum1/1 -> Dual Port RAM System3/4

== system gm_uz_mlp_three_layer/uz_mlp_three_layer/reluLayer_8Parallel1/MAC7 ==
  rd_addr : Inport  OutDataTypeStr=fixdt(0, 10, 0)  PortDimensions=1  SampleTime=1
  b : Inport  Port=2  OutDataTypeStr=fixdt(1, 32, 14)  PortDimensions=1  SampleTime=1
  axi_signals : Inport  Port=3  SampleTime=1
  fromStateMachine : Inport  Port=4  SampleTime=1
  AND : Logic  IconShape=distinctive  AllPortsSameDT=off  OutDataTypeStr=boolean
  AND1 : Logic  IconShape=distinctive  AllPortsSameDT=off  OutDataTypeStr=boolean
  Bus Selector : BusSelector  OutputSignals=axi_weightData,axi_weightAddr,axi_weightsWriteEnable,axi_biasData,axi_biasAddr,axi_biasWriteEnable,axi_layerNr
  Bus Selector1 : BusSelector  OutputSignals=endin,validIn,startin,mac_counter,write_enable,n_perceptron
  Compare To Constant : simulink/Logic and Bit Operations/Compare To Constant  relop===  const=ParallelNr  OutDataTypeStr=boolean
  Compare To Constant1 : simulink/Logic and Bit Operations/Compare To Constant  relop===  const=ParallelNr  OutDataTypeStr=boolean
  Compare To Constant2 : simulink/Logic and Bit Operations/Compare To Constant  relop===  const=LayerNr  OutDataTypeStr=boolean
  Constant : Constant  Value=nStart  OutDataTypeStr=Inherit: Inherit via back propagation  SampleTime=-1
  Dual Port RAM System1 : hdlsllib/HDL RAMs/Dual Port RAM System  RAMType=Simple dual port  WriteOutputValue=New data  RAMInitialValue=[layer.bias(nStart:nEnd);zeros(1024-length(layer.bias(nStart:nEnd)),1)]  SimulateUsing=Code generation
      settings: SourceProductBaseCode=SL
  Dual Port RAM System2 : hdlsllib/HDL RAMs/Dual Port RAM System  RAMType=Simple dual port  WriteOutputValue=New data  RAMInitialValue=[0]  SimulateUsing=Code generation
      settings: SourceProductBaseCode=SL
  Dual Port RAM System3 : hdlsllib/HDL RAMs/Dual Port RAM System  RAMType=Simple dual port  WriteOutputValue=New data  RAMInitialValue=[0;reshape(layer.weights(:,nStart:nEnd),[],1);zeros(1023-length(reshape(layer.weights(:,nStart:nEnd),[],1)),1)]  SimulateUsing=Code generation
      settings: SourceProductBaseCode=SL
  Gain : Gain  Gain=size(layer.weights(:,nStart:nEnd),1)  OutDataTypeStr=Inherit: Same as input
  Multiply-Accumulate1 : hdlsllib/HDL Operations/Multiply-Accumulate  opMode=Streaming - using Start and End ports  initValueSetting=Dialog  initValue=0  initValueSetting2=Input port  initValue2=0  initValueSetting3=Dialog  initValue3=0  num_samples=2  RndMeth2=Floor  RndMeth3=Floor  datatype2=fixdt(1,32,14)  datatype3=Inherit: Inherit via back propagation  validOut=on  endInandOut=on  startOut=on  countOut=on  dim=-1  DoSatur=off  parallel=off
      settings: SourceProductBaseCode=SL
  Saturation1 : Saturate  UpperLimit=nn_data_type_max  LowerLimit=0
  Sum : Sum  Inputs=|++  OutDataTypeStr=Inherit: Same as first input
  Sum1 : Sum  Inputs=|++  OutDataTypeStr=Inherit: Same as first input
  Terminator : Terminator
  rd_dout : Outport  SampleTime=1
  startOut : Outport  Port=2  SampleTime=1
  endOut : Outport  Port=3  SampleTime=1
  wires:
  rd_addr/1 -> Dual Port RAM System2/4
  b/1 -> Multiply-Accumulate1/2
  axi_signals/1 -> Bus Selector/1
  fromStateMachine/1 -> Bus Selector1/1
  AND/1 -> Dual Port RAM System3/3
  AND1/1 -> Dual Port RAM System1/3
  Bus Selector/1 -> Dual Port RAM System3/1
  Bus Selector/2 -> Dual Port RAM System3/2
  Bus Selector/3 -> Compare To Constant/1
  Bus Selector/4 -> Dual Port RAM System1/1
  Bus Selector/5 -> Dual Port RAM System1/2
  Bus Selector/6 -> Compare To Constant1/1
  Bus Selector/7 -> Compare To Constant2/1
  Bus Selector1/1 -> Multiply-Accumulate1/4
  Bus Selector1/2 -> Multiply-Accumulate1/5
  Bus Selector1/3 -> Multiply-Accumulate1/3
  Bus Selector1/4 -> Sum1/2
  Bus Selector1/5 -> Dual Port RAM System2/3
  Bus Selector1/6 -> Sum/1, Gain/1, Dual Port RAM System1/4
  Compare To Constant/1 -> AND/1
  Compare To Constant1/1 -> AND1/1
  Compare To Constant2/1 -> AND1/2, AND/2
  Constant/1 -> Sum/2
  Dual Port RAM System1/1 -> Multiply-Accumulate1/6
  Dual Port RAM System2/1 -> rd_dout/1
  Dual Port RAM System3/1 -> Multiply-Accumulate1/1
  Gain/1 -> Sum1/1
  Multiply-Accumulate1/1 -> Saturation1/1
  Multiply-Accumulate1/2 -> startOut/1
  Multiply-Accumulate1/3 -> endOut/1
  Multiply-Accumulate1/4 -> Terminator/1
  Saturation1/1 -> Dual Port RAM System2/1
  Sum/1 -> Dual Port RAM System2/2
  Sum1/1 -> Dual Port RAM System3/4

== system gm_uz_mlp_three_layer/uz_mlp_three_layer/reluLayer_8Parallel1/MATLAB Function1 ==
  readAddr : Inport  OutDataTypeStr=fixdt(0, 10, 0)  PortDimensions=1  SampleTime=1
  MATLAB Function1 : MATLAB Function  TreatAsAtomicUnit=on
  y : Outport  SampleTime=1
  wires:
  MATLAB Function1/1(y) -> y/1
  readAddr/1 -> MATLAB Function1/1(readAddr)

== system gm_uz_mlp_three_layer/uz_mlp_three_layer/reluLayer_8Parallel1/StateMachines1 ==
  triggerCalc : Inport  OutDataTypeStr=boolean  SampleTime=1
  mac_startOut : Inport  Port=2  OutDataTypeStr=boolean  SampleTime=1
  end_out : Inport  Port=3  OutDataTypeStr=boolean  SampleTime=1
  Bus Creator : BusCreator  Inputs=6
  Compare To Constant : simulink/Logic and Bit Operations/Compare To Constant  relop===  const=layer.weight_dimension(1)  OutDataTypeStr=boolean
  Compare To Constant1 : simulink/Logic and Bit Operations/Compare To Constant  relop===  const=layer.weight_dimension(2)/ParallelDSP-1  OutDataTypeStr=boolean
  Delay2 : Delay  DelayLength=1
  Delay3 : Delay  DelayLength=1
  Delay4 : Delay  DelayLength=1
  Detect Rise Positive : simulink/Logic and Bit Operations/Detect Rise Positive  vinit=0  OutDataTypeStr=boolean
  index_counter : hdlsllib/Sources/HDL Counter  CountType=Count limited  CountInit=1  CountStep=1  CountMax=layer.weight_dimension(1)  CountFromType=Initial value  CountFrom=1  CountResetPort=on  CountLoadPort=off  CountEnbPort=on  CountDirPort=off  CountHitOutputPort=off  CountDataType=Unsigned  CountWordLen=10  CountFracLen=0  CountSampTime=1
  layer_control : Subsystem
  mac_control : Subsystem
  perceptron_counter1 : hdlsllib/Sources/HDL Counter  CountType=Count limited  CountInit=0  CountStep=1  CountMax=layer.weight_dimension(2)/ParallelDSP-1  CountFromType=Initial value  CountFrom=0  CountResetPort=on  CountLoadPort=off  CountEnbPort=on  CountDirPort=off  CountHitOutputPort=off  CountDataType=Unsigned  CountWordLen=10  CountFracLen=0  CountSampTime=1
  mac_counter : Outport  SampleTime=1
  layer_rdy : Outport  Port=2  SampleTime=1
  layer_finished : Outport  Port=3  SampleTime=1
  toMac : Outport  Port=4  SampleTime=1
  wires:
  triggerCalc/1 -> Detect Rise Positive/1
  mac_startOut/1 -> mac_control/5(mac_startOut)
  end_out/1 -> Delay3/1, mac_control/3(end_out)
  Bus Creator/1 -> toMac/1
  Compare To Constant/1 -> mac_control/2(counter_finished)
  Compare To Constant1/1 -> layer_control/3(cnt_finished)
  Delay2/1 -> Compare To Constant/1
  Delay3/1 -> mac_control/4(end_out_delay)
  Delay4/1 -> layer_control/2(mac_ready)
  Detect Rise Positive/1 -> layer_control/1(ext_enable)
  index_counter/1 -> Bus Creator/4, Delay2/1, mac_counter/1  "mac_counter"
  layer_control/1(enable_mac) -> mac_control/1(external_enable)
  layer_control/2(layer_rdy) -> layer_rdy/1
  layer_control/3(cnt_enable) -> perceptron_counter1/2
  layer_control/4(counter_rest) -> perceptron_counter1/1
  layer_control/5(layer_finished) -> layer_finished/1
  mac_control/1(index_counter_enb) -> index_counter/2
  mac_control/2(mac_startIn) -> Bus Creator/3  "startin"
  mac_control/3(mac_endIn) -> Bus Creator/1  "endin"
  mac_control/4(mac_validIn) -> Bus Creator/2  "validIn"
  mac_control/5(index_counter_rst) -> index_counter/1
  mac_control/6(write_ram) -> Bus Creator/5  "write_enable"
  mac_control/7(mac_ready) -> Delay4/1
  perceptron_counter1/1 -> Compare To Constant1/1, Bus Creator/6  "n_perceptron"

== system gm_uz_mlp_three_layer/uz_mlp_three_layer/LastLayer/StateMachines/layer_control ==
  ext_enable : Inport  OutDataTypeStr=boolean  PortDimensions=1  SampleTime=1
  mac_ready : Inport  Port=2  OutDataTypeStr=boolean  PortDimensions=1  SampleTime=1
  cnt_finished : Inport  Port=3  OutDataTypeStr=boolean  PortDimensions=1  SampleTime=1
  layer_control : Stateflow chart  TreatAsAtomicUnit=on
  enable_mac : Outport  SampleTime=1
  layer_rdy : Outport  Port=2  SampleTime=1
  cnt_enable : Outport  Port=3  SampleTime=1
  counter_rest : Outport  Port=4  SampleTime=1
  layer_finished : Outport  Port=5  SampleTime=1
  wires:
  ext_enable/1 -> layer_control/1(ext_enable)
  mac_ready/1 -> layer_control/2(mac_ready)
  cnt_finished/1 -> layer_control/3(cnt_finished)
  layer_control/1(enable_mac) -> enable_mac/1
  layer_control/2(layer_rdy) -> layer_rdy/1
  layer_control/3(cnt_enable) -> cnt_enable/1
  layer_control/4(counter_rest) -> counter_rest/1
  layer_control/5(layer_finished) -> layer_finished/1

== system gm_uz_mlp_three_layer/uz_mlp_three_layer/LastLayer/StateMachines/mac_control ==
  external_enable : Inport  OutDataTypeStr=boolean  PortDimensions=1  SampleTime=1
  counter_finished : Inport  Port=2  OutDataTypeStr=boolean  PortDimensions=1  SampleTime=1
  end_out : Inport  Port=3  OutDataTypeStr=boolean  PortDimensions=1  SampleTime=1
  end_out_delay : Inport  Port=4  OutDataTypeStr=boolean  PortDimensions=1  SampleTime=1
  mac_startOut : Inport  Port=5  OutDataTypeStr=boolean  PortDimensions=1  SampleTime=1
  mac_control : Stateflow chart  TreatAsAtomicUnit=on
  index_counter_enb : Outport  SampleTime=1
  mac_startIn : Outport  Port=2  SampleTime=1
  mac_endIn : Outport  Port=3  SampleTime=1
  mac_validIn : Outport  Port=4  SampleTime=1
  index_counter_rst : Outport  Port=5  SampleTime=1
  write_ram : Outport  Port=6  SampleTime=1
  mac_ready : Outport  Port=7  SampleTime=1
  wires:
  external_enable/1 -> mac_control/1(external_enable)
  counter_finished/1 -> mac_control/2(counter_finished)
  end_out/1 -> mac_control/3(end_out)
  end_out_delay/1 -> mac_control/4(end_out_delay)
  mac_startOut/1 -> mac_control/5(mac_startOut)
  mac_control/1(index_counter_enb) -> index_counter_enb/1
  mac_control/2(mac_startIn) -> mac_startIn/1
  mac_control/3(mac_endIn) -> mac_endIn/1
  mac_control/4(mac_validIn) -> mac_validIn/1
  mac_control/5(index_counter_rst) -> index_counter_rst/1
  mac_control/6(write_ram) -> write_ram/1
  mac_control/7(mac_ready) -> mac_ready/1

== system gm_uz_mlp_three_layer/uz_mlp_three_layer/LastLayer/parallelOutput/holdValue ==
  takeNewValue : Inport  OutDataTypeStr=boolean  PortDimensions=1  SampleTime=1
  data : Inport  Port=2  OutDataTypeStr=fixdt(1, 32, 14)  PortDimensions=1  SampleTime=1
  Delay1 : Delay  DelayLength=1
  Switch : Switch  Criteria=u2 ~= 0
  out : Outport  SampleTime=1
  wires:
  takeNewValue/1 -> Switch/2
  data/1 -> Switch/1
  Delay1/1 -> Switch/3
  Switch/1 -> Delay1/1, out/1

== system gm_uz_mlp_three_layer/uz_mlp_three_layer/LastLayer/parallelOutput/holdValue1 ==
  takeNewValue : Inport  OutDataTypeStr=boolean  PortDimensions=1  SampleTime=1
  data : Inport  Port=2  OutDataTypeStr=fixdt(1, 32, 14)  PortDimensions=1  SampleTime=1
  Delay1 : Delay  DelayLength=1
  Switch : Switch  Criteria=u2 ~= 0
  out : Outport  SampleTime=1
  wires:
  takeNewValue/1 -> Switch/2
  data/1 -> Switch/1
  Delay1/1 -> Switch/3
  Switch/1 -> Delay1/1, out/1
